simulink model "thrustLoop"  (R2020b)
settings: Solver=VariableStepAuto  StartTime=0.0  StopTime=50  RelTol=1e-3
settings Model: Creator=bosto  LastModifiedBy=bosto

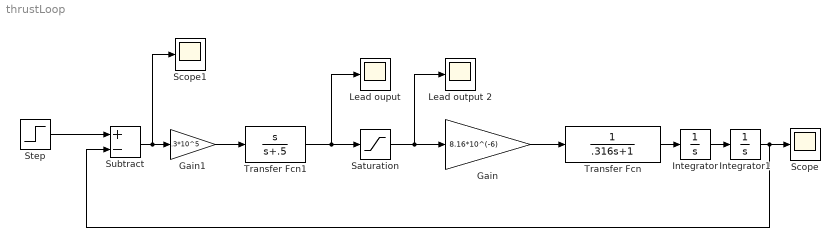
== system thrustLoop ==
  Gain : Gain  Gain=8.16*10^(-6)
  Gain1 : Gain  Gain=.3*10^5
  Integrator : Integrator
  Integrator1 : Integrator
  Lead ouput : Scope
  Lead output 2 : Scope
  Saturation : Saturate  UpperLimit=24000  LowerLimit=-40000  LinearizeAsGain=off  ZeroCross=off
  Scope : Scope
  Scope1 : Scope
  Step : Step  Time=0  SampleTime=0
  Subtract : Sum  Inputs=+-
  Transfer Fcn : TransferFcn  Denominator=[.316 1]
  Transfer Fcn1 : TransferFcn  Numerator=[1 0]  Denominator=[1 .5]
  wires:
  Gain/1 -> Transfer Fcn/1
  Subtract/1 -> Scope1/1, Gain1/1
  Transfer Fcn/1 -> Integrator/1
  Step/1 -> Subtract/1
  Integrator/1 -> Integrator1/1
  Integrator1/1 -> Subtract/2, Scope/1
  Gain1/1 -> Transfer Fcn1/1
  Transfer Fcn1/1 -> Saturation/1, Lead ouput/1
  Saturation/1 -> Lead output 2/1, Gain/1
